simulink model "P1_DevDriv_z_krancowka_2015a_good_swingup"  (R2015a)
settings: Solver=ode5  SolverMode=SingleTasking  StartTime=0.0  StopTime=999  FixedStep=0.01  RelTol=1e-3  AbsTol=1e-6
undefined symbols (not defined in the file): Cntrl, g, J, K_reg, L, M, m, RTDAC4PCIBaseAddress
libraries: simulink x8
settings Model: SimulationMode=external  CovHtmlReporting=off  CovSFcnEnable=off  ExtModeTrigDuration=12000  ExtModeTrigDurationFloating=999000  ExtModeTrigLevel=0.400000  Creator=jims  LastModifiedBy=Student
settings DataIOCC: ExternalInput=[]  InitialState=[]  LimitDataPoints=off  MaxDataPoints=5000  SignalLoggingSaveFormat=ModelDataLogs  SaveOutput=off  SaveTime=off  SignalLoggingName=sigsOut
settings OptimizationCC: BooleanDataType=off  ExpressionDepthLimit=2147483647
settings DebuggingCC: SaveWithParameterizedLinksMsg=none  UnderspecifiedInitializationDetection=Classic  MergeDetectMultiDrivingBlocksExec=none  SignalResolutionControl=TryResolveAllWithWarning  MultiTaskDSMMsg=warning  MultiTaskCondExecSysMsg=none  IntegerOverflowMsg=none  FcnCallInpInsideContextMsg=EnableAllAsWarning  StateNameClashWarn=warning  IntegerSaturationMsg=none
settings HardwareCC: ProdBitPerLong=64  ProdBitPerPointer=64  ProdIntDivRoundTo=Zero  ProdEndianess=LittleEndian  ProdWordSize=64  ProdHWDeviceType=Intel->x86-64  TargetBitPerLong=64  TargetBitPerPointer=64  TargetIntDivRoundTo=Zero  TargetEndianess=LittleEndian  TargetWordSize=64  TargetHWDeviceType=Intel->x86-64
settings RTWCC: SystemTargetFile=rtwin.tlc  TemplateMakefile=rtwin.tmf  Description=Real-Time Windows Target  RTWCompilerOptimization=on
settings CodeAppCC: MaxIdLength=95
settings TargetCC: TargetPreCompLibLocation=C:\Program Files\MATLAB\R2015aSP1\toolbox\sldrt\lib\win64

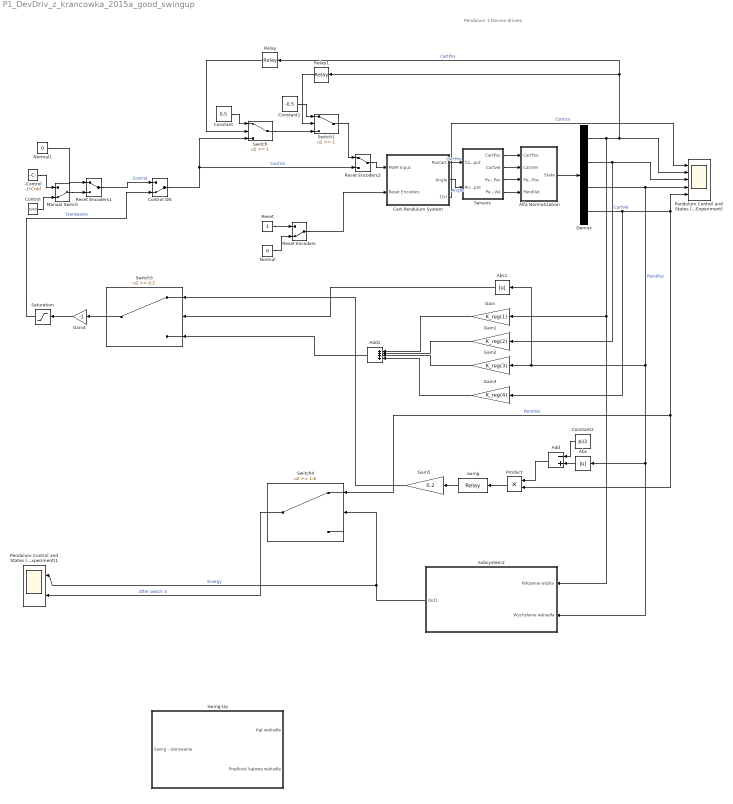
== system P1_DevDriv_z_krancowka_2015a_good_swingup ==
  note: Pendulum 1
      | Device drivers
  -Control : Constant  Value=-1*Cntrl
  Abs : Abs
  Abs1 : Abs
  Add : Sum  Inputs=-+
  Add1 : Sum  Inputs=++++
  Alfa Normalization : Subsystem  mask(Choose mode:){pos=Inverted Pendulum}
      mask prompts: pos "Choose mode:"
      mask TypeOptions pos: Inverted Pendulum | Crane Controller
  Cart-Pendulum System : Subsystem  mask{BaseAddress=RTDAC4PCIBaseAddress(-1,-1), T0=0.01}
      mask prompts: BaseAddress "Base Address:"; T0 "Sampling Period:"
      mask Display: plot( [0.725 0.725], [1.05 0.375], 0.725+0.05*sin([0:0.5:7]), 0.325+0.05*cos([0:0.5:7]), [-0.3 -0.3], [-0.3 -0.3], [1.8 1.8], [1.8 1.8], [0.1 1.4], [0.95 0.95], [0.1 1.4], [0.92 0.92], [0.65 0.8], [1 1], [0.65 0.8], [1.1 1.1], [0.65 0.65], [1.1 1], [0.8 0.8], [1 1.1] )
  Constant : Constant  Value=0.5
  Constant1 : Constant  Value=-0.5
  Constant2 : Constant  Value=pi/2
  Control : Constant  Value=Cntrl
  Control ON : ManualSwitch  CurrentSetting=0
  Demux : Demux
  Gain : Gain  Gain=K_reg(1)
  Gain1 : Gain  Gain=K_reg(2)
  Gain2 : Gain  Gain=K_reg(3)
  Gain3 : Gain  Gain=K_reg(4)
  Gain4 : Gain  Gain=-1
  Gain5 : Gain  Gain=0.2
  Manual Switch : ManualSwitch  CurrentSetting=0
  Normal : Constant  Value=0
  Normal1 : Constant  Value=0
  Pendulum Control and States (Experiment) : Scope  NumInputPorts=5
      settings: TimeRange=100  YMin=-1~-0.0988519~-10~3.13392~0  YMax=1~-0.0988519~0~3.13392~2000  SaveName=P1_ExpData  MaxDataPoints=50000
  Pendulum Control and States (Experiment)1 : Scope  NumInputPorts=2
      settings: TimeRange=100  YMin=-1~-175000  YMax=12~175000  SaveName=P1_ExpData1  MaxDataPoints=50000
  Product : Product
  Relay : Relay  OnSwitchValue=0.7  OffSwitchValue=0.6
  Relay1 : Relay  OnSwitchValue=-0.6  OffSwitchValue=-0.7  OnOutputValue=0  OffOutputValue=1
  Reset : Constant
  Reset Encoders : ManualSwitch  CurrentSetting=0
  Reset Encoders1 : ManualSwitch
  Reset Encoders2 : ManualSwitch
  Saturation : Saturate  UpperLimit=1  LowerLimit=-1
  Sensors : Subsystem  mask(PENDULUM Output){T0=0.01}
      mask prompts: T0 "Sample Time"
      mask help: PCL-812 PG Device Driver
  Subsystem2 : Subsystem
  Swing-Up : Subsystem
  Switch : Switch  Threshold=1
  Switch1 : Switch  Threshold=1
  Switch3 : Switch  Threshold=0.2
  Switch4 : Switch  Threshold=1.6
  swing : Relay  OffOutputValue=-1
  wires:
  Reset Encoders/1 -> Cart-Pendulum System/2(Reset Encoders)
  Sensors/3(PendPos) -> Alfa Normalization/3(PendPos)
  Sensors/4(PendVel) -> Alfa Normalization/4(PendVel)
  Sensors/1(CartPos) -> Alfa Normalization/1(CartPos)
  Sensors/2(CartVel) -> Alfa Normalization/2(CartVel)
  Demux/1 -> Subsystem2/1(Położenie wózka), Gain/1, Pendulum Control and States (Experiment)/2, Relay/1, Relay1/1  "CartPos"
  Demux/2 -> Gain1/1, Pendulum Control and States (Experiment)/3  "CartVel"
  Demux/3 -> Abs/1, Subsystem2/2(Wychylenie wahadła), Abs1/1, Gain2/1, Pendulum Control and States (Experiment)/4  "PendPos"
  Demux/4 -> Gain3/1, Product/2, Switch4/1, Pendulum Control and States (Experiment)/5  "PendVel"
  Cart-Pendulum System/1(PosCart) -> Sensors/1(CartPosInput)  "CartPos"
  Cart-Pendulum System/2(Angle) -> Sensors/2(AngleInput)  "Angle"
  Normal/1 -> Reset Encoders/2
  Reset/1 -> Reset Encoders/1
  Normal1/1 -> Reset Encoders1/1
  Manual Switch/1 -> Reset Encoders1/2
  Control/1 -> Manual Switch/2
  -Control/1 -> Manual Switch/1
  Control ON/1 -> Reset Encoders2/2, Switch/3  "Control"
  Relay/1 -> Switch/2
  Constant/1 -> Switch/1
  Reset Encoders2/1 -> Cart-Pendulum System/1(PWM Input)
  Relay1/1 -> Switch1/2
  Constant1/1 -> Switch1/1
  Switch/1 -> Switch1/3
  Switch1/1 -> Reset Encoders2/1
  Gain/1 -> Add1/1
  Gain1/1 -> Add1/2
  Gain2/1 -> Add1/3
  Gain3/1 -> Add1/4
  Gain4/1 -> Saturation/1
  Reset Encoders1/1 -> Control ON/1  "Control"
  Abs1/1 -> Switch3/2
  Alfa Normalization/1(State) -> Demux/1
  Cart-Pendulum System/3(Ctrl) -> Pendulum Control and States (Experiment)/1  "Control"
  Subsystem2/1(Out1) -> Switch4/2, Pendulum Control and States (Experiment)1/1  "Energy"
  Switch4/1 -> Pendulum Control and States (Experiment)1/2  "After switch 4"
  Switch3/1 -> Gain4/1
  Add1/1 -> Switch3/3
  Saturation/1 -> Control ON/2  "Sterowanie"
  Constant2/1 -> Add/1
  Abs/1 -> Add/2
  Add/1 -> Product/1
  Product/1 -> swing/1
  swing/1 -> Gain5/1
  Gain5/1 -> Switch3/1

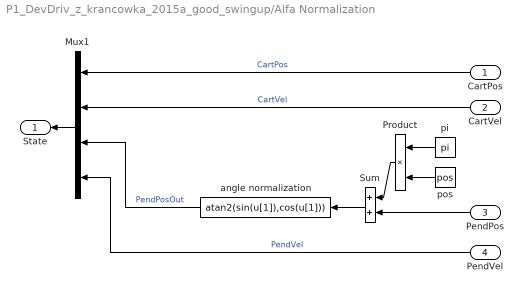
== system P1_DevDriv_z_krancowka_2015a_good_swingup/Alfa Normalization ==
  CartPos : Inport
  CartVel : Inport  Port=2
  PendPos : Inport  Port=3
  PendVel : Inport  Port=4
  Mux1 : Mux
  Product : Product  SaturateOnIntegerOverflow=on  InputSameDT=on  OutDataTypeStr=Inherit: Same as first input
  Sum : Sum  SaturateOnIntegerOverflow=on  InputSameDT=on  OutDataTypeStr=Inherit: Same as first input
  angle normalization : Fcn  Expr=atan2(sin(u[1]),cos(u[1]))
  pi : Constant  Value=pi
  pos : Constant  Value=pos
  State : Outport  InitialOutput=0
  wires:
  angle normalization/1 -> Mux1/3  "PendPosOut"
  PendVel/1 -> Mux1/4  "PendVel"
  CartVel/1 -> Mux1/2  "CartVel"
  CartPos/1 -> Mux1/1  "CartPos"
  Mux1/1 -> State/1
  Sum/1 -> angle normalization/1
  PendPos/1 -> Sum/2
  pi/1 -> Product/1
  pos/1 -> Product/2
  Product/1 -> Sum/1

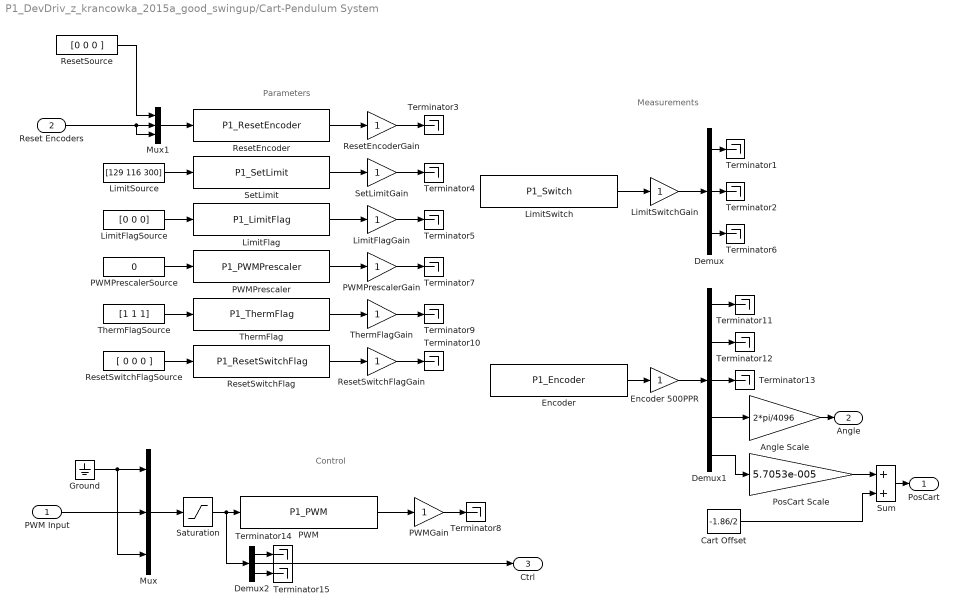
== system P1_DevDriv_z_krancowka_2015a_good_swingup/Cart-Pendulum System ==
  note: Measurements
  note: Control
  note: Parameters
  PWM Input : Inport
  Reset Encoders : Inport  Port=2
  Angle Scale : Gain  Gain=2*pi/4096  OutDataTypeStr=Inherit: Same as input  ParamDataTypeStr=Inherit: Same as input
  Cart Offset : Constant  Value=-1.86/2
  Demux : Demux  Outputs=3
  Demux1 : Demux  Outputs=5
  Demux2 : Demux  Outputs=3
  Encoder : S-Function  FunctionName=P1_Encoder  Parameters=BaseAddress, T0
  Encoder 500PPR : Gain  SaturateOnIntegerOverflow=on  OutDataTypeStr=Inherit: Same as input  ParamDataTypeStr=Inherit: Same as input
  Ground : Ground
  LimitFlag : S-Function  FunctionName=P1_LimitFlag  Parameters=BaseAddress, T0
  LimitFlagGain : Gain  SaturateOnIntegerOverflow=on  OutDataTypeStr=Inherit: Same as input  ParamDataTypeStr=Inherit: Same as input
  LimitFlagSource : Constant  Value=[0 0 0]
  LimitSource : Constant  Value=[129 116 300]
  LimitSwitch : S-Function  FunctionName=P1_Switch  Parameters=BaseAddress, T0
  LimitSwitchGain : Gain  SaturateOnIntegerOverflow=on  OutDataTypeStr=Inherit: Same as input  ParamDataTypeStr=Inherit: Same as input
  Mux : Mux  Inputs=3
  Mux1 : Mux  Inputs=[3 1 1]
  PWM : S-Function  FunctionName=P1_PWM  Parameters=BaseAddress, T0
  PWMGain : Gain  SaturateOnIntegerOverflow=on  OutDataTypeStr=Inherit: Same as input  ParamDataTypeStr=Inherit: Same as input
  PWMPrescaler : S-Function  FunctionName=P1_PWMPrescaler  Parameters=BaseAddress, T0
  PWMPrescalerGain : Gain  SaturateOnIntegerOverflow=on  OutDataTypeStr=Inherit: Same as input  ParamDataTypeStr=Inherit: Same as input
  PWMPrescalerSource : Constant  Value=0
  PosCart Scale : Gain  Gain=5.7053e-005  OutDataTypeStr=Inherit: Same as input  ParamDataTypeStr=Inherit: Same as input
  ResetEncoder : S-Function  FunctionName=P1_ResetEncoder  Parameters=BaseAddress, T0
  ResetEncoderGain : Gain  SaturateOnIntegerOverflow=on  OutDataTypeStr=Inherit: Same as input  ParamDataTypeStr=Inherit: Same as input
  ResetSource : Constant  Value=[0 0 0 ]
  "ResetSwitchFlag " : S-Function  FunctionName=P1_ResetSwitchFlag  Parameters=BaseAddress, T0
  ResetSwitchFlagGain : Gain  SaturateOnIntegerOverflow=on  OutDataTypeStr=Inherit: Same as input  ParamDataTypeStr=Inherit: Same as input
  ResetSwitchFlagSource : Constant  Value=[ 0 0 0 ]
  Saturation : Saturate
  SetLimit : S-Function  FunctionName=P1_SetLimit  Parameters=BaseAddress, T0
  SetLimitGain : Gain  SaturateOnIntegerOverflow=on  OutDataTypeStr=Inherit: Same as input  ParamDataTypeStr=Inherit: Same as input
  Sum : Sum  SaturateOnIntegerOverflow=on  InputSameDT=on  OutDataTypeStr=Inherit: Same as first input
  Terminator{1..15} (15 alike) : Terminator
  "ThermFlag " : S-Function  FunctionName=P1_ThermFlag  Parameters=BaseAddress, T0
  ThermFlagGain : Gain  SaturateOnIntegerOverflow=on  OutDataTypeStr=Inherit: Same as input  ParamDataTypeStr=Inherit: Same as input
  ThermFlagSource : Constant  Value=[1 1 1]
  PosCart : Outport  InitialOutput=0
  Angle : Outport  Port=2  InitialOutput=0
  Ctrl : Outport  Port=3  InitialOutput=0
  wires:
  Demux1/1 -> Terminator11/1
  Demux1/2 -> Terminator12/1
  Demux1/3 -> Terminator13/1
  Demux1/4 -> Angle Scale/1
  Demux1/5 -> PosCart Scale/1
  Angle Scale/1 -> Angle/1
  Demux/3 -> Terminator6/1
  Demux/2 -> Terminator2/1
  Demux/1 -> Terminator1/1
  LimitSwitchGain/1 -> Demux/1
  LimitSwitch/1 -> LimitSwitchGain/1
  Ground/1 -> Mux/1, Mux/3
  PWM Input/1 -> Mux/2
  ResetSwitchFlagGain/1 -> Terminator10/1
  ThermFlagGain/1 -> Terminator9/1
  PWMPrescalerGain/1 -> Terminator7/1
  LimitFlagGain/1 -> Terminator5/1
  SetLimitGain/1 -> Terminator4/1
  ResetEncoderGain/1 -> Terminator3/1
  ResetSwitchFlagSource/1 -> "ResetSwitchFlag "/1
  ThermFlagSource/1 -> "ThermFlag "/1
  PWMPrescalerSource/1 -> PWMPrescaler/1
  LimitFlagSource/1 -> LimitFlag/1
  LimitSource/1 -> SetLimit/1
  "ResetSwitchFlag "/1 -> ResetSwitchFlagGain/1
  "ThermFlag "/1 -> ThermFlagGain/1
  PWMPrescaler/1 -> PWMPrescalerGain/1
  LimitFlag/1 -> LimitFlagGain/1
  SetLimit/1 -> SetLimitGain/1
  ResetEncoder/1 -> ResetEncoderGain/1
  PWM/1 -> PWMGain/1
  Mux/1 -> Saturation/1
  Saturation/1 -> Demux2/1, PWM/1
  Encoder/1 -> Encoder 500PPR/1
  Encoder 500PPR/1 -> Demux1/1
  Mux1/1 -> ResetEncoder/1
  ResetSource/1 -> Mux1/1
  Reset Encoders/1 -> Mux1/2, Mux1/3
  PosCart Scale/1 -> Sum/1
  Sum/1 -> PosCart/1
  Cart Offset/1 -> Sum/2
  PWMGain/1 -> Terminator8/1
  Demux2/2 -> Ctrl/1
  Demux2/1 -> Terminator14/1
  Demux2/3 -> Terminator15/1

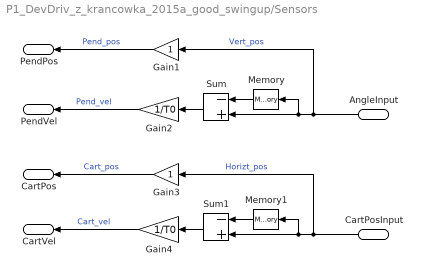
== system P1_DevDriv_z_krancowka_2015a_good_swingup/Sensors ==
  CartPosInput : Inport
  AngleInput : Inport  Port=2
  Gain1 : Gain  SaturateOnIntegerOverflow=on  OutDataTypeStr=Inherit: Same as input  ParamDataTypeStr=Inherit: Same as input
  Gain2 : Gain  Gain=1/T0  SaturateOnIntegerOverflow=on  OutDataTypeStr=Inherit: Same as input  ParamDataTypeStr=Inherit: Same as input
  Gain3 : Gain  SaturateOnIntegerOverflow=on  OutDataTypeStr=Inherit: Same as input  ParamDataTypeStr=Inherit: Same as input
  Gain4 : Gain  Gain=1/T0  SaturateOnIntegerOverflow=on  OutDataTypeStr=Inherit: Same as input  ParamDataTypeStr=Inherit: Same as input
  Memory : Memory
  Memory1 : Memory
  Sum : Sum  Inputs=-+  SaturateOnIntegerOverflow=on  InputSameDT=on  OutDataTypeStr=Inherit: Same as first input
  Sum1 : Sum  Inputs=-+  SaturateOnIntegerOverflow=on  InputSameDT=on  OutDataTypeStr=Inherit: Same as first input
  CartPos : Outport  InitialOutput=0
  CartVel : Outport  Port=2  InitialOutput=0
  PendPos : Outport  Port=3  InitialOutput=0
  PendVel : Outport  Port=4  InitialOutput=0
  wires:
  Gain4/1 -> CartVel/1  "Cart_vel"
  Sum1/1 -> Gain4/1
  Memory1/1 -> Sum1/1
  Sum/1 -> Gain2/1
  Memory/1 -> Sum/1
  CartPosInput/1 -> Memory1/1, Sum1/2, Gain3/1  "Horizt_pos"
  AngleInput/1 -> Memory/1, Sum/2, Gain1/1  "Vert_pos"
  Gain2/1 -> PendVel/1  "Pend_vel"
  Gain1/1 -> PendPos/1  "Pend_pos"
  Gain3/1 -> CartPos/1  "Cart_pos"

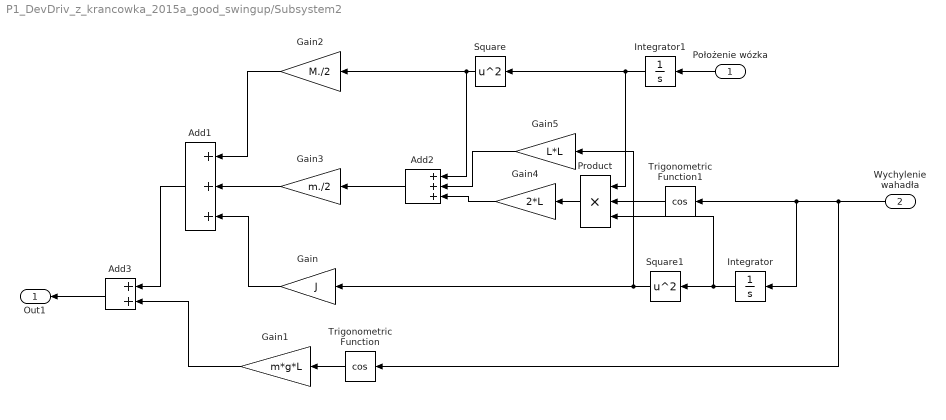
== system P1_DevDriv_z_krancowka_2015a_good_swingup/Subsystem2 ==
  Położenie wózka : Inport
  Wychylenie wahadła : Inport  Port=2
  Add1 : Sum  Inputs=+++
  Add2 : Sum  Inputs=+++
  Add3 : Sum
  Gain : Gain  Gain=J
  Gain1 : Gain  Gain=m*g*L
  Gain2 : Gain  Gain=M./2
  Gain3 : Gain  Gain=m./2
  Gain4 : Gain  Gain=2*L
  Gain5 : Gain  Gain=L*L
  Integrator : Integrator
  Integrator1 : Integrator
  Product : Product  Inputs=3
  Square : Math  Operator=square  SaturateOnIntegerOverflow=on
  Square1 : Math  Operator=square  SaturateOnIntegerOverflow=on
  Trigonometric Function : Trigonometry  Operator=cos
  Trigonometric Function1 : Trigonometry  Operator=cos
  Out1 : Outport
  wires:
  Trigonometric Function/1 -> Gain1/1
  Gain1/1 -> Add3/2
  Gain/1 -> Add1/3
  Add3/1 -> Out1/1
  Wychylenie wahadła/1 -> Trigonometric Function/1, Trigonometric Function1/1, Integrator/1
  Gain2/1 -> Add1/1
  Square/1 -> Add2/1, Gain2/1
  Gain3/1 -> Add1/2
  Add2/1 -> Gain3/1
  Gain4/1 -> Add2/3
  Gain5/1 -> Add2/2
  Product/1 -> Gain4/1
  Trigonometric Function1/1 -> Product/2
  Integrator1/1 -> Square/1, Product/1
  Położenie wózka/1 -> Integrator1/1
  Add1/1 -> Add3/1
  Integrator/1 -> Product/3, Square1/1
  Square1/1 -> Gain5/1, Gain/1

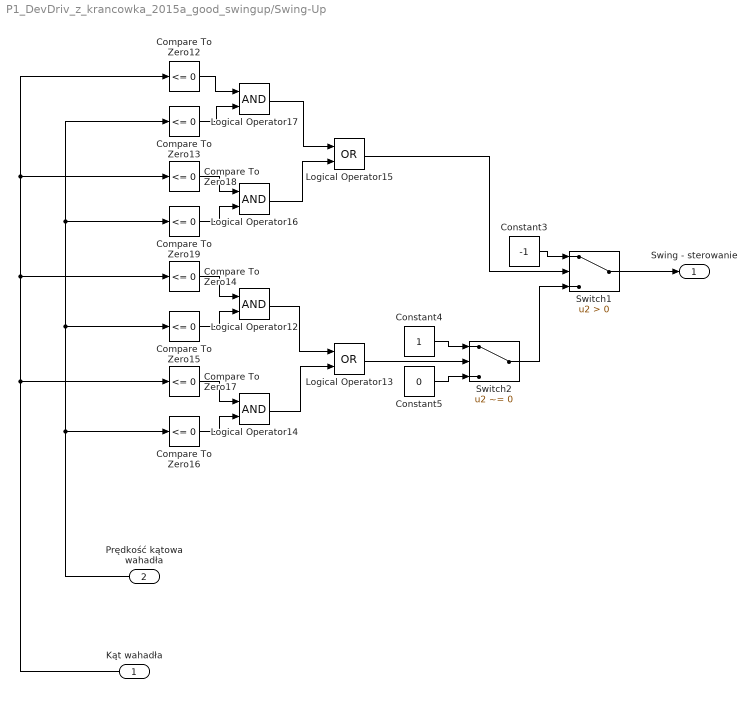
== system P1_DevDriv_z_krancowka_2015a_good_swingup/Swing-Up ==
  Kąt wahadła : Inport
  Prędkość kątowa wahadła : Inport  Port=2
  Compare To Zero{12..19} (8 alike) : simulink/Logic and Bit Operations/Compare To Zero  relop=<=  OutDataTypeStr=boolean
  Constant3 : Constant  Value=-1
  Constant4 : Constant
  Constant5 : Constant  Value=0
  Logical Operator{12,14,16..17} (4 alike) : Logic  AllPortsSameDT=off  OutDataTypeStr=boolean
  Logical Operator13 : Logic  Operator=OR  AllPortsSameDT=off  OutDataTypeStr=boolean
  Logical Operator15 : Logic  Operator=OR  AllPortsSameDT=off  OutDataTypeStr=boolean
  Switch1 : Switch  Criteria=u2 > Threshold
  Switch2 : Switch  Criteria=u2 ~= 0
  Swing - sterowanie : Outport
  wires:
  Prędkość kątowa wahadła/1 -> Compare To Zero15/1, Compare To Zero19/1, Compare To Zero13/1, Compare To Zero16/1
  Kąt wahadła/1 -> Compare To Zero17/1, Compare To Zero14/1, Compare To Zero18/1, Compare To Zero12/1
  Switch1/1 -> Swing - sterowanie/1
  Compare To Zero16/1 -> Logical Operator14/2
  Compare To Zero18/1 -> Logical Operator16/1
  Switch2/1 -> Switch1/3
  Logical Operator14/1 -> Logical Operator13/2
  Constant5/1 -> Switch2/3
  Logical Operator12/1 -> Logical Operator13/1
  Compare To Zero17/1 -> Logical Operator14/1
  Compare To Zero12/1 -> Logical Operator17/1
  Logical Operator16/1 -> Logical Operator15/2
  Compare To Zero14/1 -> Logical Operator12/1
  Constant4/1 -> Switch2/1
  Compare To Zero15/1 -> Logical Operator12/2
  Compare To Zero13/1 -> Logical Operator17/2
  Logical Operator17/1 -> Logical Operator15/1
  Logical Operator15/1 -> Switch1/2
  Constant3/1 -> Switch1/1
  Compare To Zero19/1 -> Logical Operator16/2
  Logical Operator13/1 -> Switch2/2
